simulink model "atrias_HW_boom_nmSt_kinSw_v2"  (R2015a)
settings: Solver=ode4  StartTime=0.0  StopTime=inf  FixedStep=sample_time  RelTol=1e-3
values from neighbouring files (symbols this model uses):
  control_start_time = 15    [setParams.m]
  flag_CtrlMode = 0    [setParams.m]
  kinSw_alpha_start = 130*pi/180    (= 2.26892802759)    [setParams.m]
  kinSw_alpha_tgt = 70*pi/180    (= 1.2217304764)    [setParams.m]
  kinSw_t_start = 0.5    [setParams.m]
  poser_LLegAlp = (initial_l_leg_angle -pi/2)*180/pi    (= 105)    [setParams.m]
  poser_LLegLen = initial_l_leg_length    (= 0.8)    [setParams.m]
  poser_RLegAlp = (initial_r_leg_angle -pi/2)*180/pi    (= 75)    [setParams.m]
  poser_RLegLen = initial_r_leg_length    (= 0.8)    [setParams.m]
  tune_kinSw_alpha_start = kinSw_alpha_start*180/pi    (= 130)    [setParams.m]
  tune_kinSw_alpha_tgt = kinSw_alpha_tgt*180/pi    (= 70)    [setParams.m]
  tune_kinSw_len_min = kinSw_len_min    (= 0.6)    [setParams.m]
  tune_kinSw_len_tgt = kinSw_len_tgt    (= 0.9)    [setParams.m]
  tune_M1_G = 9.5    [setParams.m]
  tune_M3_0 = CtrlPar_theta0*180/pi    [setParams.m]
  tune_M3_D = St_GainDTh_HFL*5    [setParams.m]
  tune_M3_P = St_GainTh_HFL*5    [setParams.m]
undefined symbols (not defined in the file or in its folder): A1_notch_f1, A2_notch_f1, A_kalman_fourbar_gear, A_lpf_dtau, B1_lpf_dtau, B1_notch_f1, B2_lpf_dtau, B2_notch_f1, B_kalman_fourbar_gear, boom_mount_angle, boom_mount_to_center_diagonal, c_jointstop, C_kalman_fourbar_gear, contactThr, d_vertical_com, delta_phi_max, delta_phi_max_buffer, delta_phi_max_dropoff, delta_phi_min, Discrete, FmaxBFSH, FmaxGLU, FmaxHAM, FmaxHFL, FmaxRF, FmaxVAS, FPCtrlPar, g, gain_nodes_sea_torque, HIP_MTR_MAX_CONT_TORQUE, initial_dx_estimate, j_motor, k_leg_spring, K_notch_f1, k_sea, kalman_load_to_deflect_transmission, kd_lateral, kd_motor, kd_shin_max, kd_shin_min, kd_splay_max, kd_splay_min, kd_thigh_max, kd_thigh_min, kp_lateral, kp_motor, kp_sea_torque, kp_shin_max, kp_shin_min, kp_splay_max, kp_splay_min, kp_thigh_max, kp_thigh_min, l_boom, l_seg, l_v, lateral_motor_efficiency, lateral_offset, lateral_target_angle_right, lateral_transition_force ... (+124)
libraries: simulink_extras x27, simulink x11, ctrlSharedLib x4
(part 4 of 8)

== system atrias_HW_boom_nmSt_kinSw_v2/Control/Behavior Control/Virtual Neuromuscular Control/Muscle Layer/GLU1 ==
  note: SOLEUS Muscle-Tendon Dynamics
  note: Excitation Contraction Coupling
  STIM : Inport
  lmtc [m] : Inport  Port=2
  1 : Product  Inputs=**  SaturateOnIntegerOverflow=on  InputSameDT=on  OutDataTypeStr=Inherit: Same as first input
  1/lslack : Gain  Gain=1/lslackGLU  SaturateOnIntegerOverflow=on  OutDataTypeStr=Inherit: Same as input  ParamDataTypeStr=Inherit: Same as input
  BE force-length relation : Subsystem
  CE force-length relation : Subsystem
  CE inverse force-velocity relation : Subsystem
  Constant : Constant  Value=lslackGLU
  ECC TransferFcn : simulink_extras/Additional Linear/Transfer Fcn (with initial outputs)  N=[1]  D="[mtu_tau  1]"  Y0=mtu_preA  U0=0
      settings: AttributesFormatString=pre-activation: %<Y0>
  Fmax : Gain  Gain=FmaxGLU  SaturateOnIntegerOverflow=on  OutDataTypeStr=Inherit: Same as input  ParamDataTypeStr=Inherit: Same as input
  Fv = Fse / (A*Fce) : Product  Inputs=*/  SaturateOnIntegerOverflow=on  InputSameDT=on  OutDataTypeStr=Inherit: Same as first input
  Integrator : Integrator  InitialConditionSource=external  LowerSaturationLimit=0.05
  PE force-length relation : Subsystem
  SE force-length relation : Subsystem
  Saturation : Saturate  UpperLimit=1  LowerLimit=0.01
  Sum : Sum  Inputs=|+-  SaturateOnIntegerOverflow=on  InputSameDT=on  OutDataTypeStr=Inherit: Same as first input
  Sum2 : Sum  Inputs=|-+  SaturateOnIntegerOverflow=on  InputSameDT=on  OutDataTypeStr=Inherit: Same as first input
  Sum3 : Sum  SaturateOnIntegerOverflow=on  InputSameDT=on  OutDataTypeStr=Inherit: Same as first input
  Sum4 : Sum  SaturateOnIntegerOverflow=on  InputSameDT=on  OutDataTypeStr=Inherit: Same as first input
  lce/lopt : Gain  Gain=1/loptGLU  SaturateOnIntegerOverflow=on  OutDataTypeStr=Inherit: Same as input  ParamDataTypeStr=Inherit: Same as input
  vmax*lopt : Gain  Gain=vmaxGLU*loptGLU  SaturateOnIntegerOverflow=on  OutDataTypeStr=Inherit: Same as input  ParamDataTypeStr=Inherit: Same as input
  Fmtc : Outport  InitialOutput=0
  Lce : Outport  Port=2  InitialOutput=0
  Vce : Outport  Port=3  InitialOutput=0
  A : Outport  Port=4  InitialOutput=0
  wires:
  Integrator/1 -> Sum/2, lce/lopt/1, Lce/1  "lce"
  Sum/1 -> 1/lslack/1  "lse"
  lce/lopt/1 -> CE force-length relation/1(lce [lopt]), BE force-length relation/1(lce [lopt]), PE force-length relation/1(lce [lopt])
  Fv = Fse / (A*Fce)/1 -> CE inverse force-velocity relation/1(Fv[Fmax])  "fv"
  vmax*lopt/1 -> Integrator/1, Vce/1  "vce"
  lmtc [m]/1 -> Sum2/2, Sum/1  "lmtc"
  Fmax/1 -> Fmtc/1  "Fmtc"
  1/lslack/1 -> SE force-length relation/1(lse [lslack])
  SE force-length relation/1(fse [Fmax]) -> Fmax/1, Sum4/1
  Sum2/1 -> Integrator/2
  Constant/1 -> Sum2/1
  CE force-length relation/1(fce [Fmax]) -> 1/1
  Sum4/1 -> Fv = Fse / (A*Fce)/1
  PE force-length relation/1(fpe [Fmax]) -> Sum3/1
  1/1 -> Sum3/2
  BE force-length relation/1(fbe [Fmax]) -> Sum4/2
  Sum3/1 -> Fv = Fse / (A*Fce)/2
  CE inverse force-velocity relation/1(v[vmax]) -> vmax*lopt/1
  STIM/1 -> ECC TransferFcn/1
  ECC TransferFcn/1 -> Saturation/1
  Saturation/1 -> A/1, 1/2

== system atrias_HW_boom_nmSt_kinSw_v2/Control/Behavior Control/Virtual Neuromuscular Control/Muscle Layer/HAM ==
  note: SOLEUS Muscle-Tendon Dynamics
  note: Excitation Contraction Coupling
  STIM : Inport
  lmtc [m] : Inport  Port=2
  1 : Product  Inputs=**  SaturateOnIntegerOverflow=on  InputSameDT=on  OutDataTypeStr=Inherit: Same as first input
  1/lslack : Gain  Gain=1/lslackHAM  SaturateOnIntegerOverflow=on  OutDataTypeStr=Inherit: Same as input  ParamDataTypeStr=Inherit: Same as input
  BE force-length relation : Subsystem
  CE force-length relation : Subsystem
  CE inverse force-velocity relation : Subsystem
  Constant : Constant  Value=lslackHAM
  ECC TransferFcn : simulink_extras/Additional Linear/Transfer Fcn (with initial outputs)  N=[1]  D="[mtu_tau  1]"  Y0=mtu_preA  U0=0
      settings: AttributesFormatString=pre-activation: %<Y0>
  Fmax : Gain  Gain=FmaxHAM  SaturateOnIntegerOverflow=on  OutDataTypeStr=Inherit: Same as input  ParamDataTypeStr=Inherit: Same as input
  Fv = Fse / (A*Fce) : Product  Inputs=*/  SaturateOnIntegerOverflow=on  InputSameDT=on  OutDataTypeStr=Inherit: Same as first input
  Integrator : Integrator  InitialConditionSource=external  LowerSaturationLimit=0.05
  PE force-length relation : Subsystem
  SE force-length relation : Subsystem
  Saturation : Saturate  UpperLimit=1  LowerLimit=0.01
  Sum : Sum  Inputs=|+-  SaturateOnIntegerOverflow=on  InputSameDT=on  OutDataTypeStr=Inherit: Same as first input
  Sum2 : Sum  Inputs=|-+  SaturateOnIntegerOverflow=on  InputSameDT=on  OutDataTypeStr=Inherit: Same as first input
  Sum3 : Sum  SaturateOnIntegerOverflow=on  InputSameDT=on  OutDataTypeStr=Inherit: Same as first input
  Sum4 : Sum  SaturateOnIntegerOverflow=on  InputSameDT=on  OutDataTypeStr=Inherit: Same as first input
  lce/lopt : Gain  Gain=1/loptHAM  SaturateOnIntegerOverflow=on  OutDataTypeStr=Inherit: Same as input  ParamDataTypeStr=Inherit: Same as input
  vmax*lopt : Gain  Gain=vmaxHAM*loptHAM  SaturateOnIntegerOverflow=on  OutDataTypeStr=Inherit: Same as input  ParamDataTypeStr=Inherit: Same as input
  Fmtc : Outport  InitialOutput=0
  Lce : Outport  Port=2  InitialOutput=0
  Vce : Outport  Port=3  InitialOutput=0
  A : Outport  Port=4  InitialOutput=0
  wires:
  Integrator/1 -> Sum/2, lce/lopt/1, Lce/1  "lce"
  Sum/1 -> 1/lslack/1  "lse"
  lce/lopt/1 -> CE force-length relation/1(lce [lopt]), BE force-length relation/1(lce [lopt]), PE force-length relation/1(lce [lopt])
  Fv = Fse / (A*Fce)/1 -> CE inverse force-velocity relation/1(Fv[Fmax])  "fv"
  vmax*lopt/1 -> Integrator/1, Vce/1  "vce"
  lmtc [m]/1 -> Sum2/2, Sum/1  "lmtc"
  Fmax/1 -> Fmtc/1  "Fmtc"
  1/lslack/1 -> SE force-length relation/1(lse [lslack])
  SE force-length relation/1(fse [Fmax]) -> Fmax/1, Sum4/1
  Sum2/1 -> Integrator/2
  Constant/1 -> Sum2/1
  CE force-length relation/1(fce [Fmax]) -> 1/1
  Sum4/1 -> Fv = Fse / (A*Fce)/1
  PE force-length relation/1(fpe [Fmax]) -> Sum3/1
  1/1 -> Sum3/2
  BE force-length relation/1(fbe [Fmax]) -> Sum4/2
  Sum3/1 -> Fv = Fse / (A*Fce)/2
  CE inverse force-velocity relation/1(v[vmax]) -> vmax*lopt/1
  STIM/1 -> ECC TransferFcn/1
  ECC TransferFcn/1 -> Saturation/1
  Saturation/1 -> A/1, 1/2

== system atrias_HW_boom_nmSt_kinSw_v2/Control/Behavior Control/Virtual Neuromuscular Control/Muscle Layer/HAM Link ==
  note: HAM Attachment
  phi34 [rad] : Inport
  phi23 [rad] : Inport  Port=2
  Constant1 : Constant  Value=rHAMk
  Constant2 : Constant  Value=phirefHAMk
  Constant3 : Constant  Value=rHAMh
  Constant4 : Constant  Value=lslackHAM+loptHAM
  Constant5 : Constant  Value=phirefHAMh
  Gain2 : Gain  Gain=rhoHAMh
  Gain4 : Gain  Gain=rhoHAMk
  Product : Product  RndMeth=Zero
  Product1 : Product  RndMeth=Zero
  Sum1 : Sum  Inputs=|+-
  Sum4 : Sum  Inputs=|+-
  Sum5 : Sum  Inputs=-++
  lmtu [m] : Outport
  lever34 [m] : Outport  Port=2
  lever23 [m] : Outport  Port=3
  wires:
  Sum5/1 -> lmtu [m]/1
  Constant4/1 -> Sum5/2
  Gain4/1 -> Sum5/3
  Gain2/1 -> Sum5/1
  phi34 [rad]/1 -> Sum4/1
  Constant5/1 -> Sum4/2
  Sum4/1 -> Product/1
  Constant3/1 -> Product/2, lever34 [m]/1
  Product/1 -> Gain2/1
  phi23 [rad]/1 -> Sum1/1
  Constant2/1 -> Sum1/2
  Sum1/1 -> Product1/1
  Constant1/1 -> Product1/2, lever23 [m]/1
  Product1/1 -> Gain4/1

== system atrias_HW_boom_nmSt_kinSw_v2/Control/Behavior Control/Virtual Neuromuscular Control/Muscle Layer/HAM Link1 ==
  note: HAM Attachment
  phi34 [rad] : Inport
  phi23 [rad] : Inport  Port=2
  Constant1 : Constant  Value=rHAMk
  Constant2 : Constant  Value=phirefHAMk
  Constant3 : Constant  Value=rHAMh
  Constant4 : Constant  Value=lslackHAM+loptHAM
  Constant5 : Constant  Value=phirefHAMh
  Gain2 : Gain  Gain=rhoHAMh
  Gain4 : Gain  Gain=rhoHAMk
  Product : Product  RndMeth=Zero
  Product1 : Product  RndMeth=Zero
  Sum1 : Sum  Inputs=|+-
  Sum4 : Sum  Inputs=|+-
  Sum5 : Sum  Inputs=-++
  lmtu [m] : Outport
  lever34 [m] : Outport  Port=2
  lever23 [m] : Outport  Port=3
  wires:
  Sum5/1 -> lmtu [m]/1
  Constant4/1 -> Sum5/2
  Gain4/1 -> Sum5/3
  Gain2/1 -> Sum5/1
  phi34 [rad]/1 -> Sum4/1
  Constant5/1 -> Sum4/2
  Sum4/1 -> Product/1
  Constant3/1 -> Product/2, lever34 [m]/1
  Product/1 -> Gain2/1
  phi23 [rad]/1 -> Sum1/1
  Constant2/1 -> Sum1/2
  Sum1/1 -> Product1/1
  Constant1/1 -> Product1/2, lever23 [m]/1
  Product1/1 -> Gain4/1

== system atrias_HW_boom_nmSt_kinSw_v2/Control/Behavior Control/Virtual Neuromuscular Control/Muscle Layer/HAM1 ==
  note: SOLEUS Muscle-Tendon Dynamics
  note: Excitation Contraction Coupling
  STIM : Inport
  lmtc [m] : Inport  Port=2
  1 : Product  Inputs=**  SaturateOnIntegerOverflow=on  InputSameDT=on  OutDataTypeStr=Inherit: Same as first input
  1/lslack : Gain  Gain=1/lslackHAM  SaturateOnIntegerOverflow=on  OutDataTypeStr=Inherit: Same as input  ParamDataTypeStr=Inherit: Same as input
  BE force-length relation : Subsystem
  CE force-length relation : Subsystem
  CE inverse force-velocity relation : Subsystem
  Constant : Constant  Value=lslackHAM
  ECC TransferFcn : simulink_extras/Additional Linear/Transfer Fcn (with initial outputs)  N=[1]  D="[mtu_tau  1]"  Y0=mtu_preA  U0=0
      settings: AttributesFormatString=pre-activation: %<Y0>
  Fmax : Gain  Gain=FmaxHAM  SaturateOnIntegerOverflow=on  OutDataTypeStr=Inherit: Same as input  ParamDataTypeStr=Inherit: Same as input
  Fv = Fse / (A*Fce) : Product  Inputs=*/  SaturateOnIntegerOverflow=on  InputSameDT=on  OutDataTypeStr=Inherit: Same as first input
  Integrator : Integrator  InitialConditionSource=external  LowerSaturationLimit=0.05
  PE force-length relation : Subsystem
  SE force-length relation : Subsystem
  Saturation : Saturate  UpperLimit=1  LowerLimit=0.01
  Sum : Sum  Inputs=|+-  SaturateOnIntegerOverflow=on  InputSameDT=on  OutDataTypeStr=Inherit: Same as first input
  Sum2 : Sum  Inputs=|-+  SaturateOnIntegerOverflow=on  InputSameDT=on  OutDataTypeStr=Inherit: Same as first input
  Sum3 : Sum  SaturateOnIntegerOverflow=on  InputSameDT=on  OutDataTypeStr=Inherit: Same as first input
  Sum4 : Sum  SaturateOnIntegerOverflow=on  InputSameDT=on  OutDataTypeStr=Inherit: Same as first input
  lce/lopt : Gain  Gain=1/loptHAM  SaturateOnIntegerOverflow=on  OutDataTypeStr=Inherit: Same as input  ParamDataTypeStr=Inherit: Same as input
  vmax*lopt : Gain  Gain=vmaxHAM*loptHAM  SaturateOnIntegerOverflow=on  OutDataTypeStr=Inherit: Same as input  ParamDataTypeStr=Inherit: Same as input
  Fmtc : Outport  InitialOutput=0
  Lce : Outport  Port=2  InitialOutput=0
  Vce : Outport  Port=3  InitialOutput=0
  A : Outport  Port=4  InitialOutput=0
  wires:
  Integrator/1 -> Sum/2, lce/lopt/1, Lce/1  "lce"
  Sum/1 -> 1/lslack/1  "lse"
  lce/lopt/1 -> CE force-length relation/1(lce [lopt]), BE force-length relation/1(lce [lopt]), PE force-length relation/1(lce [lopt])
  Fv = Fse / (A*Fce)/1 -> CE inverse force-velocity relation/1(Fv[Fmax])  "fv"
  vmax*lopt/1 -> Integrator/1, Vce/1  "vce"
  lmtc [m]/1 -> Sum2/2, Sum/1  "lmtc"
  Fmax/1 -> Fmtc/1  "Fmtc"
  1/lslack/1 -> SE force-length relation/1(lse [lslack])
  SE force-length relation/1(fse [Fmax]) -> Fmax/1, Sum4/1
  Sum2/1 -> Integrator/2
  Constant/1 -> Sum2/1
  CE force-length relation/1(fce [Fmax]) -> 1/1
  Sum4/1 -> Fv = Fse / (A*Fce)/1
  PE force-length relation/1(fpe [Fmax]) -> Sum3/1
  1/1 -> Sum3/2
  BE force-length relation/1(fbe [Fmax]) -> Sum4/2
  Sum3/1 -> Fv = Fse / (A*Fce)/2
  CE inverse force-velocity relation/1(v[vmax]) -> vmax*lopt/1
  STIM/1 -> ECC TransferFcn/1
  ECC TransferFcn/1 -> Saturation/1
  Saturation/1 -> A/1, 1/2

== system atrias_HW_boom_nmSt_kinSw_v2/Control/Behavior Control/Virtual Neuromuscular Control/Muscle Layer/HFL ==
  note: SOLEUS Muscle-Tendon Dynamics
  note: Excitation Contraction Coupling
  STIM : Inport
  lmtc [m] : Inport  Port=2
  1 : Product  Inputs=**  SaturateOnIntegerOverflow=on  InputSameDT=on  OutDataTypeStr=Inherit: Same as first input
  1/lslack : Gain  Gain=1/lslackHFL  SaturateOnIntegerOverflow=on  OutDataTypeStr=Inherit: Same as input  ParamDataTypeStr=Inherit: Same as input
  BE force-length relation : Subsystem
  CE force-length relation : Subsystem
  CE inverse force-velocity relation : Subsystem
  Constant : Constant  Value=lslackHFL
  ECC TransferFcn : simulink_extras/Additional Linear/Transfer Fcn (with initial outputs)  N=[1]  D="[mtu_tau  1]"  Y0=mtu_preA  U0=0
      settings: AttributesFormatString=pre-activation: %<Y0>
  Fmax : Gain  Gain=FmaxHFL  SaturateOnIntegerOverflow=on  OutDataTypeStr=Inherit: Same as input  ParamDataTypeStr=Inherit: Same as input
  Fv = Fse / (A*Fce) : Product  Inputs=*/  SaturateOnIntegerOverflow=on  InputSameDT=on  OutDataTypeStr=Inherit: Same as first input
  Integrator : Integrator  InitialConditionSource=external  LowerSaturationLimit=0.05
  PE force-length relation : Subsystem
  SE force-length relation : Subsystem
  Saturation : Saturate  UpperLimit=1  LowerLimit=0.01
  Sum : Sum  Inputs=|+-  SaturateOnIntegerOverflow=on  InputSameDT=on  OutDataTypeStr=Inherit: Same as first input
  Sum2 : Sum  Inputs=|-+  SaturateOnIntegerOverflow=on  InputSameDT=on  OutDataTypeStr=Inherit: Same as first input
  Sum3 : Sum  SaturateOnIntegerOverflow=on  InputSameDT=on  OutDataTypeStr=Inherit: Same as first input
  Sum4 : Sum  SaturateOnIntegerOverflow=on  InputSameDT=on  OutDataTypeStr=Inherit: Same as first input
  lce/lopt : Gain  Gain=1/loptHFL  SaturateOnIntegerOverflow=on  OutDataTypeStr=Inherit: Same as input  ParamDataTypeStr=Inherit: Same as input
  vmax*lopt : Gain  Gain=vmaxHFL*loptHFL  SaturateOnIntegerOverflow=on  OutDataTypeStr=Inherit: Same as input  ParamDataTypeStr=Inherit: Same as input
  Fmtc : Outport  InitialOutput=0
  Lce : Outport  Port=2  InitialOutput=0
  Vce : Outport  Port=3  InitialOutput=0
  A : Outport  Port=4  InitialOutput=0
  wires:
  Integrator/1 -> Sum/2, lce/lopt/1, Lce/1  "lce"
  Sum/1 -> 1/lslack/1  "lse"
  lce/lopt/1 -> CE force-length relation/1(lce [lopt]), BE force-length relation/1(lce [lopt]), PE force-length relation/1(lce [lopt])
  Fv = Fse / (A*Fce)/1 -> CE inverse force-velocity relation/1(Fv[Fmax])  "fv"
  vmax*lopt/1 -> Integrator/1, Vce/1  "vce"
  lmtc [m]/1 -> Sum2/2, Sum/1  "lmtc"
  Fmax/1 -> Fmtc/1  "Fmtc"
  1/lslack/1 -> SE force-length relation/1(lse [lslack])
  SE force-length relation/1(fse [Fmax]) -> Fmax/1, Sum4/1
  Sum2/1 -> Integrator/2
  Constant/1 -> Sum2/1
  CE force-length relation/1(fce [Fmax]) -> 1/1
  Sum4/1 -> Fv = Fse / (A*Fce)/1
  PE force-length relation/1(fpe [Fmax]) -> Sum3/1
  1/1 -> Sum3/2
  BE force-length relation/1(fbe [Fmax]) -> Sum4/2
  Sum3/1 -> Fv = Fse / (A*Fce)/2
  CE inverse force-velocity relation/1(v[vmax]) -> vmax*lopt/1
  STIM/1 -> ECC TransferFcn/1
  ECC TransferFcn/1 -> Saturation/1
  Saturation/1 -> A/1, 1/2

== system atrias_HW_boom_nmSt_kinSw_v2/Control/Behavior Control/Virtual Neuromuscular Control/Muscle Layer/HFL Link ==
  note: HFL Attachment
  phi34 [rad] : Inport
  Constant : Constant  Value=lslackHFL+loptHFL
  Constant1 : Constant  Value=rHFL
  Constant2 : Constant  Value=phirefHFL
  Gain2 : Gain  Gain=rhoHFL
  Product : Product  RndMeth=Zero
  Sum2 : Sum  Inputs=|+-
  Sum5 : Sum  Inputs=|++
  lmtu [m] : Outport
  lever [m] : Outport  Port=2
  wires:
  Constant/1 -> Sum5/1
  Sum5/1 -> lmtu [m]/1
  Product/1 -> Gain2/1
  phi34 [rad]/1 -> Sum2/1
  Constant2/1 -> Sum2/2
  Sum2/1 -> Product/1
  Constant1/1 -> Product/2, lever [m]/1
  Gain2/1 -> Sum5/2

== system atrias_HW_boom_nmSt_kinSw_v2/Control/Behavior Control/Virtual Neuromuscular Control/Muscle Layer/HFL Link1 ==
  note: HFL Attachment
  phi34 [rad] : Inport
  Constant : Constant  Value=lslackHFL+loptHFL
  Constant1 : Constant  Value=rHFL
  Constant2 : Constant  Value=phirefHFL
  Gain2 : Gain  Gain=rhoHFL
  Product : Product  RndMeth=Zero
  Sum2 : Sum  Inputs=|+-
  Sum5 : Sum  Inputs=|++
  lmtu [m] : Outport
  lever [m] : Outport  Port=2
  wires:
  Constant/1 -> Sum5/1
  Sum5/1 -> lmtu [m]/1
  Product/1 -> Gain2/1
  phi34 [rad]/1 -> Sum2/1
  Constant2/1 -> Sum2/2
  Sum2/1 -> Product/1
  Constant1/1 -> Product/2, lever [m]/1
  Gain2/1 -> Sum5/2

== system atrias_HW_boom_nmSt_kinSw_v2/Control/Behavior Control/Virtual Neuromuscular Control/Muscle Layer/HFL1 ==
  note: SOLEUS Muscle-Tendon Dynamics
  note: Excitation Contraction Coupling
  STIM : Inport
  lmtc [m] : Inport  Port=2
  1 : Product  Inputs=**  SaturateOnIntegerOverflow=on  InputSameDT=on  OutDataTypeStr=Inherit: Same as first input
  1/lslack : Gain  Gain=1/lslackHFL  SaturateOnIntegerOverflow=on  OutDataTypeStr=Inherit: Same as input  ParamDataTypeStr=Inherit: Same as input
  BE force-length relation : Subsystem
  CE force-length relation : Subsystem
  CE inverse force-velocity relation : Subsystem
  Constant : Constant  Value=lslackHFL
  ECC TransferFcn : simulink_extras/Additional Linear/Transfer Fcn (with initial outputs)  N=[1]  D="[mtu_tau  1]"  Y0=mtu_preA  U0=0
      settings: AttributesFormatString=pre-activation: %<Y0>
  Fmax : Gain  Gain=FmaxHFL  SaturateOnIntegerOverflow=on  OutDataTypeStr=Inherit: Same as input  ParamDataTypeStr=Inherit: Same as input
  Fv = Fse / (A*Fce) : Product  Inputs=*/  SaturateOnIntegerOverflow=on  InputSameDT=on  OutDataTypeStr=Inherit: Same as first input
  Integrator : Integrator  InitialConditionSource=external  LowerSaturationLimit=0.05
  PE force-length relation : Subsystem
  SE force-length relation : Subsystem
  Saturation : Saturate  UpperLimit=1  LowerLimit=0.01
  Sum : Sum  Inputs=|+-  SaturateOnIntegerOverflow=on  InputSameDT=on  OutDataTypeStr=Inherit: Same as first input
  Sum2 : Sum  Inputs=|-+  SaturateOnIntegerOverflow=on  InputSameDT=on  OutDataTypeStr=Inherit: Same as first input
  Sum3 : Sum  SaturateOnIntegerOverflow=on  InputSameDT=on  OutDataTypeStr=Inherit: Same as first input
  Sum4 : Sum  SaturateOnIntegerOverflow=on  InputSameDT=on  OutDataTypeStr=Inherit: Same as first input
  lce/lopt : Gain  Gain=1/loptHFL  SaturateOnIntegerOverflow=on  OutDataTypeStr=Inherit: Same as input  ParamDataTypeStr=Inherit: Same as input
  vmax*lopt : Gain  Gain=vmaxHFL*loptHFL  SaturateOnIntegerOverflow=on  OutDataTypeStr=Inherit: Same as input  ParamDataTypeStr=Inherit: Same as input
  Fmtc : Outport  InitialOutput=0
  Lce : Outport  Port=2  InitialOutput=0
  Vce : Outport  Port=3  InitialOutput=0
  A : Outport  Port=4  InitialOutput=0
  wires:
  Integrator/1 -> Sum/2, lce/lopt/1, Lce/1  "lce"
  Sum/1 -> 1/lslack/1  "lse"
  lce/lopt/1 -> CE force-length relation/1(lce [lopt]), BE force-length relation/1(lce [lopt]), PE force-length relation/1(lce [lopt])
  Fv = Fse / (A*Fce)/1 -> CE inverse force-velocity relation/1(Fv[Fmax])  "fv"
  vmax*lopt/1 -> Integrator/1, Vce/1  "vce"
  lmtc [m]/1 -> Sum2/2, Sum/1  "lmtc"
  Fmax/1 -> Fmtc/1  "Fmtc"
  1/lslack/1 -> SE force-length relation/1(lse [lslack])
  SE force-length relation/1(fse [Fmax]) -> Fmax/1, Sum4/1
  Sum2/1 -> Integrator/2
  Constant/1 -> Sum2/1
  CE force-length relation/1(fce [Fmax]) -> 1/1
  Sum4/1 -> Fv = Fse / (A*Fce)/1
  PE force-length relation/1(fpe [Fmax]) -> Sum3/1
  1/1 -> Sum3/2
  BE force-length relation/1(fbe [Fmax]) -> Sum4/2
  Sum3/1 -> Fv = Fse / (A*Fce)/2
  CE inverse force-velocity relation/1(v[vmax]) -> vmax*lopt/1
  STIM/1 -> ECC TransferFcn/1
  ECC TransferFcn/1 -> Saturation/1
  Saturation/1 -> A/1, 1/2

== system atrias_HW_boom_nmSt_kinSw_v2/Control/Behavior Control/Virtual Neuromuscular Control/Muscle Layer/L BFSH Link ==
  note: BFSH Attachment
  phi23 [rad] : Inport
  Constant : Constant  Value=lslackBFSH+loptBFSH
  Constant1 : Constant  Value=rBFSH
  Constant2 : Constant  Value=phirefBFSH
  Gain4 : Gain  Gain=rhoBFSH
  Product : Product  RndMeth=Zero
  Sum2 : Sum  Inputs=|+-
  Sum5 : Sum  Inputs=|++
  lmtu [m] : Outport
  lever [m] : Outport  Port=2
  wires:
  Constant/1 -> Sum5/1
  Sum5/1 -> lmtu [m]/1
  Gain4/1 -> Sum5/2
  Product/1 -> Gain4/1
  phi23 [rad]/1 -> Sum2/1
  Constant2/1 -> Sum2/2
  Sum2/1 -> Product/1
  Constant1/1 -> Product/2, lever [m]/1

== system atrias_HW_boom_nmSt_kinSw_v2/Control/Behavior Control/Virtual Neuromuscular Control/Muscle Layer/L BFSH Link1 ==
  note: BFSH Attachment
  phi23 [rad] : Inport
  Constant : Constant  Value=lslackBFSH+loptBFSH
  Constant1 : Constant  Value=rBFSH
  Constant2 : Constant  Value=phirefBFSH
  Gain4 : Gain  Gain=rhoBFSH
  Product : Product  RndMeth=Zero
  Sum2 : Sum  Inputs=|+-
  Sum5 : Sum  Inputs=|++
  lmtu [m] : Outport
  lever [m] : Outport  Port=2
  wires:
  Constant/1 -> Sum5/1
  Sum5/1 -> lmtu [m]/1
  Gain4/1 -> Sum5/2
  Product/1 -> Gain4/1
  phi23 [rad]/1 -> Sum2/1
  Constant2/1 -> Sum2/2
  Sum2/1 -> Product/1
  Constant1/1 -> Product/2, lever [m]/1

== system atrias_HW_boom_nmSt_kinSw_v2/Control/Behavior Control/Virtual Neuromuscular Control/Muscle Layer/L Hip Joint Limits ==
  note: Hip Joint Limits
  phi [rad]1 : Inport
  dphi [rad/s]1 : Inport  Port=2
  Constant : Constant  Value=0
  Gain1 : Gain  Gain=c_jointstop
  Gain5 : Gain  Gain=-1
  Gain6 : Gain  Gain=c_jointstop
  Gain7 : Gain  Gain=1/w_max_jointstop
  Manual Switch : ManualSwitch
  Mux1 : Mux  Inputs=2
  Mux2 : Mux  Inputs=2
  Overextension Torque1 : Fcn  Expr="- u(1)  *  (1-u(2)) * (u(2)<1) * (u(1)>0)"
  Overflexion Torque : Fcn  Expr="- u(1)  *  (1-u(2)) * (u(2)<1) * (u(1)<0)"
  Sum1 : Sum  Inputs=|+-
  Sum2 : Sum  Inputs=|+-
  Sum3 : Sum
  overextension angle1 : Constant  Value=phi23_max
  overflexion angle : Constant  Value=phi23_min
  M_stop [Nm]1 : Outport
  wires:
  Mux2/1 -> Overextension Torque1/1
  Gain6/1 -> Mux2/1
  dphi [rad/s]1/1 -> Gain7/1
  overextension angle1/1 -> Sum1/2
  phi [rad]1/1 -> Sum1/1, Sum2/1
  Sum1/1 -> Gain6/1
  Gain7/1 -> Gain5/1, Mux1/2
  Gain1/1 -> Mux1/1
  Sum2/1 -> Gain1/1
  overflexion angle/1 -> Sum2/2
  Mux1/1 -> Overflexion Torque/1
  Gain5/1 -> Mux2/2
  Overflexion Torque/1 -> Sum3/2
  Overextension Torque1/1 -> Sum3/1
  Sum3/1 -> Manual Switch/1
  Constant/1 -> Manual Switch/2
  Manual Switch/1 -> M_stop [Nm]1/1

== system atrias_HW_boom_nmSt_kinSw_v2/Control/Behavior Control/Virtual Neuromuscular Control/Muscle Layer/L Hip Joint Limits1 ==
  note: Hip Joint Limits
  phi [rad]1 : Inport
  dphi [rad/s]1 : Inport  Port=2
  Constant : Constant  Value=0
  Gain1 : Gain  Gain=c_jointstop
  Gain5 : Gain  Gain=-1
  Gain6 : Gain  Gain=c_jointstop
  Gain7 : Gain  Gain=1/w_max_jointstop
  Manual Switch : ManualSwitch
  Mux1 : Mux  Inputs=2
  Mux2 : Mux  Inputs=2
  Overextension Torque1 : Fcn  Expr="- u(1)  *  (1-u(2)) * (u(2)<1) * (u(1)>0)"
  Overflexion Torque : Fcn  Expr="- u(1)  *  (1-u(2)) * (u(2)<1) * (u(1)<0)"
  Sum1 : Sum  Inputs=|+-
  Sum2 : Sum  Inputs=|+-
  Sum3 : Sum
  overextension angle1 : Constant  Value=phi23_max
  overflexion angle : Constant  Value=phi23_min
  M_stop [Nm]1 : Outport
  wires:
  Mux2/1 -> Overextension Torque1/1
  Gain6/1 -> Mux2/1
  dphi [rad/s]1/1 -> Gain7/1
  overextension angle1/1 -> Sum1/2
  phi [rad]1/1 -> Sum1/1, Sum2/1
  Sum1/1 -> Gain6/1
  Gain7/1 -> Gain5/1, Mux1/2
  Gain1/1 -> Mux1/1
  Sum2/1 -> Gain1/1
  overflexion angle/1 -> Sum2/2
  Mux1/1 -> Overflexion Torque/1
  Gain5/1 -> Mux2/2
  Overflexion Torque/1 -> Sum3/2
  Overextension Torque1/1 -> Sum3/1
  Sum3/1 -> Manual Switch/1
  Constant/1 -> Manual Switch/2
  Manual Switch/1 -> M_stop [Nm]1/1

== system atrias_HW_boom_nmSt_kinSw_v2/Control/Behavior Control/Virtual Neuromuscular Control/Muscle Layer/L Knee Joint Limits ==
  note: Knee Joint Limits
  phi [rad]1 : Inport
  dphi [rad/s]1 : Inport  Port=2
  Constant : Constant  Value=0
  Gain1 : Gain  Gain=c_jointstop
  Gain5 : Gain  Gain=-1
  Gain6 : Gain  Gain=c_jointstop
  Gain7 : Gain  Gain=1/w_max_jointstop
  Manual Switch : ManualSwitch
  Mux1 : Mux  Inputs=2
  Mux2 : Mux  Inputs=2
  Overextension Torque1 : Fcn  Expr="- u(1)  *  (1-u(2)) * (u(2)<1) * (u(1)>0)"
  Overflexion Torque : Fcn  Expr="- u(1)  *  (1-u(2)) * (u(2)<1) * (u(1)<0)"
  Sum1 : Sum  Inputs=|+-
  Sum2 : Sum  Inputs=|+-
  Sum3 : Sum
  overextension angle1 : Constant  Value=phi12_max
  overflexion angle : Constant  Value=phi12_min
  M_stop [Nm]1 : Outport
  wires:
  Mux2/1 -> Overextension Torque1/1
  Gain6/1 -> Mux2/1
  dphi [rad/s]1/1 -> Gain7/1
  overextension angle1/1 -> Sum1/2
  phi [rad]1/1 -> Sum1/1, Sum2/1
  Sum1/1 -> Gain6/1
  Gain7/1 -> Gain5/1, Mux1/2
  Gain1/1 -> Mux1/1
  Sum2/1 -> Gain1/1
  overflexion angle/1 -> Sum2/2
  Mux1/1 -> Overflexion Torque/1
  Gain5/1 -> Mux2/2
  Overflexion Torque/1 -> Sum3/2
  Overextension Torque1/1 -> Sum3/1
  Sum3/1 -> Manual Switch/1
  Constant/1 -> Manual Switch/2
  Manual Switch/1 -> M_stop [Nm]1/1

== system atrias_HW_boom_nmSt_kinSw_v2/Control/Behavior Control/Virtual Neuromuscular Control/Muscle Layer/L Knee Joint Limits1 ==
  note: Knee Joint Limits
  phi [rad]1 : Inport
  dphi [rad/s]1 : Inport  Port=2
  Constant : Constant  Value=0
  Gain1 : Gain  Gain=c_jointstop
  Gain5 : Gain  Gain=-1
  Gain6 : Gain  Gain=c_jointstop
  Gain7 : Gain  Gain=1/w_max_jointstop
  Manual Switch : ManualSwitch
  Mux1 : Mux  Inputs=2
  Mux2 : Mux  Inputs=2
  Overextension Torque1 : Fcn  Expr="- u(1)  *  (1-u(2)) * (u(2)<1) * (u(1)>0)"
  Overflexion Torque : Fcn  Expr="- u(1)  *  (1-u(2)) * (u(2)<1) * (u(1)<0)"
  Sum1 : Sum  Inputs=|+-
  Sum2 : Sum  Inputs=|+-
  Sum3 : Sum
  overextension angle1 : Constant  Value=phi12_max
  overflexion angle : Constant  Value=phi12_min
  M_stop [Nm]1 : Outport
  wires:
  Mux2/1 -> Overextension Torque1/1
  Gain6/1 -> Mux2/1
  dphi [rad/s]1/1 -> Gain7/1
  overextension angle1/1 -> Sum1/2
  phi [rad]1/1 -> Sum1/1, Sum2/1
  Sum1/1 -> Gain6/1
  Gain7/1 -> Gain5/1, Mux1/2
  Gain1/1 -> Mux1/1
  Sum2/1 -> Gain1/1
  overflexion angle/1 -> Sum2/2
  Mux1/1 -> Overflexion Torque/1
  Gain5/1 -> Mux2/2
  Overflexion Torque/1 -> Sum3/2
  Overextension Torque1/1 -> Sum3/1
  Sum3/1 -> Manual Switch/1
  Constant/1 -> Manual Switch/2
  Manual Switch/1 -> M_stop [Nm]1/1

== system atrias_HW_boom_nmSt_kinSw_v2/Control/Behavior Control/Virtual Neuromuscular Control/Muscle Layer/RF ==
  note: SOLEUS Muscle-Tendon Dynamics
  note: Excitation Contraction Coupling
  STIM : Inport
  lmtc [m] : Inport  Port=2
  1 : Product  Inputs=**  SaturateOnIntegerOverflow=on  InputSameDT=on  OutDataTypeStr=Inherit: Same as first input
  1/lslack : Gain  Gain=1/lslackRF  SaturateOnIntegerOverflow=on  OutDataTypeStr=Inherit: Same as input  ParamDataTypeStr=Inherit: Same as input
  BE force-length relation : Subsystem
  CE force-length relation : Subsystem
  CE inverse force-velocity relation : Subsystem
  Constant : Constant  Value=lslackRF
  ECC TransferFcn : simulink_extras/Additional Linear/Transfer Fcn (with initial outputs)  N=[1]  D="[mtu_tau  1]"  Y0=mtu_preA  U0=0
      settings: AttributesFormatString=pre-activation: %<Y0>
  Fmax : Gain  Gain=FmaxRF  SaturateOnIntegerOverflow=on  OutDataTypeStr=Inherit: Same as input  ParamDataTypeStr=Inherit: Same as input
  Fv = Fse / (A*Fce) : Product  Inputs=*/  SaturateOnIntegerOverflow=on  InputSameDT=on  OutDataTypeStr=Inherit: Same as first input
  Integrator : Integrator  InitialConditionSource=external  LowerSaturationLimit=0.05
  PE force-length relation : Subsystem
  SE force-length relation : Subsystem
  Saturation : Saturate  UpperLimit=1  LowerLimit=0.01
  Sum : Sum  Inputs=|+-  SaturateOnIntegerOverflow=on  InputSameDT=on  OutDataTypeStr=Inherit: Same as first input
  Sum2 : Sum  Inputs=|-+  SaturateOnIntegerOverflow=on  InputSameDT=on  OutDataTypeStr=Inherit: Same as first input
  Sum3 : Sum  SaturateOnIntegerOverflow=on  InputSameDT=on  OutDataTypeStr=Inherit: Same as first input
  Sum4 : Sum  SaturateOnIntegerOverflow=on  InputSameDT=on  OutDataTypeStr=Inherit: Same as first input
  lce/lopt : Gain  Gain=1/loptRF  SaturateOnIntegerOverflow=on  OutDataTypeStr=Inherit: Same as input  ParamDataTypeStr=Inherit: Same as input
  vmax*lopt : Gain  Gain=vmaxRF*loptRF  SaturateOnIntegerOverflow=on  OutDataTypeStr=Inherit: Same as input  ParamDataTypeStr=Inherit: Same as input
  Fmtc : Outport  InitialOutput=0
  Lce : Outport  Port=2  InitialOutput=0
  Vce : Outport  Port=3  InitialOutput=0
  A : Outport  Port=4  InitialOutput=0
  wires:
  Integrator/1 -> Sum/2, lce/lopt/1, Lce/1  "lce"
  Sum/1 -> 1/lslack/1  "lse"
  lce/lopt/1 -> CE force-length relation/1(lce [lopt]), BE force-length relation/1(lce [lopt]), PE force-length relation/1(lce [lopt])
  Fv = Fse / (A*Fce)/1 -> CE inverse force-velocity relation/1(Fv[Fmax])  "fv"
  vmax*lopt/1 -> Integrator/1, Vce/1  "vce"
  lmtc [m]/1 -> Sum2/2, Sum/1  "lmtc"
  Fmax/1 -> Fmtc/1  "Fmtc"
  1/lslack/1 -> SE force-length relation/1(lse [lslack])
  SE force-length relation/1(fse [Fmax]) -> Fmax/1, Sum4/1
  Sum2/1 -> Integrator/2
  Constant/1 -> Sum2/1
  CE force-length relation/1(fce [Fmax]) -> 1/1
  Sum4/1 -> Fv = Fse / (A*Fce)/1
  PE force-length relation/1(fpe [Fmax]) -> Sum3/1
  1/1 -> Sum3/2
  BE force-length relation/1(fbe [Fmax]) -> Sum4/2
  Sum3/1 -> Fv = Fse / (A*Fce)/2
  CE inverse force-velocity relation/1(v[vmax]) -> vmax*lopt/1
  STIM/1 -> ECC TransferFcn/1
  ECC TransferFcn/1 -> Saturation/1
  Saturation/1 -> A/1, 1/2

== system atrias_HW_boom_nmSt_kinSw_v2/Control/Behavior Control/Virtual Neuromuscular Control/Muscle Layer/RF Link ==
  note: RF Attachment
  phi34 [rad] : Inport
  phi23 [rad] : Inport  Port=2
  Constant1 : Constant  Value=phimaxRFk
  Constant2 : Constant  Value=phirefRFk
  Constant3 : Constant  Value=rRFh
  Constant4 : Constant  Value=lslackRF+loptRF
  Constant5 : Constant  Value=phirefRFh
  Demux : Demux  Outputs=2
  Display : Display
  Gain1 : Gain  Gain=rRFkmax
  Gain2 : Gain  Gain=rhoRFh
  Gain3 : Gain  Gain=phiScaleRFk
  Gain4 : Gain  Gain=rhoRFk/phiScaleRFk
  Gain5 : Gain  Gain=phiScaleRFk
  Mux : Mux  Inputs=2
  Product : Product  RndMeth=Zero
  Sum1 : Sum  Inputs=-+
  Sum2 : Sum  Inputs=|+-
  Sum3 : Sum  Inputs=-+|
  Sum4 : Sum  Inputs=|+-
  Sum5 : Sum  Inputs=++-
  length change term : Trigonometry
  offset correction term : Trigonometry
  variable lever term : Trigonometry  Operator=cos
  lmtu [m] : Outport
  lever34 [m] : Outport  Port=2
  lever23 [m] : Outport  Port=3
  wires:
  Sum5/1 -> Display/1, lmtu [m]/1
  Constant4/1 -> Sum5/2
  Gain4/1 -> Sum5/3
  Gain2/1 -> Sum5/1
  phi34 [rad]/1 -> Sum4/1
  Constant5/1 -> Sum4/2
  Sum4/1 -> Product/1
  Constant3/1 -> Product/2, lever34 [m]/1
  Product/1 -> Gain2/1
  phi23 [rad]/1 -> Sum3/2
  Sum3/1 -> Gain3/1
  Constant1/1 -> Sum3/1, Sum2/2
  Sum2/1 -> Gain5/1
  Constant2/1 -> Sum2/1
  length change term/1 -> Sum1/2
  offset correction term/1 -> Sum1/1
  Sum1/1 -> Mux/1
  variable lever term/1 -> Mux/2
  Mux/1 -> Gain1/1
  Gain1/1 -> Demux/1
  Demux/2 -> lever23 [m]/1
  Demux/1 -> Gain4/1
  Gain3/1 -> variable lever term/1, length change term/1
  Gain5/1 -> offset correction term/1

== system atrias_HW_boom_nmSt_kinSw_v2/Control/Behavior Control/Virtual Neuromuscular Control/Muscle Layer/RF Link1 ==
  note: RF Attachment
  phi34 [rad] : Inport
  phi23 [rad] : Inport  Port=2
  Constant1 : Constant  Value=phimaxRFk
  Constant2 : Constant  Value=phirefRFk
  Constant3 : Constant  Value=rRFh
  Constant4 : Constant  Value=lslackRF+loptRF
  Constant5 : Constant  Value=phirefRFh
  Demux : Demux  Outputs=2
  Gain1 : Gain  Gain=rRFkmax
  Gain2 : Gain  Gain=rhoRFh
  Gain3 : Gain  Gain=phiScaleRFk
  Gain4 : Gain  Gain=rhoRFk/phiScaleRFk
  Gain5 : Gain  Gain=phiScaleRFk
  Mux : Mux  Inputs=2
  Product : Product  RndMeth=Zero
  Sum1 : Sum  Inputs=-+
  Sum2 : Sum  Inputs=|+-
  Sum3 : Sum  Inputs=-+|
  Sum4 : Sum  Inputs=|+-
  Sum5 : Sum  Inputs=++-
  length change term : Trigonometry
  offset correction term : Trigonometry
  variable lever term : Trigonometry  Operator=cos
  lmtu [m] : Outport
  lever34 [m] : Outport  Port=2
  lever23 [m] : Outport  Port=3
  wires:
  Sum5/1 -> lmtu [m]/1
  Constant4/1 -> Sum5/2
  Gain4/1 -> Sum5/3
  Gain2/1 -> Sum5/1
  phi34 [rad]/1 -> Sum4/1
  Constant5/1 -> Sum4/2
  Sum4/1 -> Product/1
  Constant3/1 -> Product/2, lever34 [m]/1
  Product/1 -> Gain2/1
  phi23 [rad]/1 -> Sum3/2
  Sum3/1 -> Gain3/1
  Constant1/1 -> Sum3/1, Sum2/2
  Sum2/1 -> Gain5/1
  Constant2/1 -> Sum2/1
  length change term/1 -> Sum1/2
  offset correction term/1 -> Sum1/1
  Sum1/1 -> Mux/1
  variable lever term/1 -> Mux/2
  Mux/1 -> Gain1/1
  Gain1/1 -> Demux/1
  Demux/2 -> lever23 [m]/1
  Demux/1 -> Gain4/1
  Gain3/1 -> variable lever term/1, length change term/1
  Gain5/1 -> offset correction term/1

== system atrias_HW_boom_nmSt_kinSw_v2/Control/Behavior Control/Virtual Neuromuscular Control/Muscle Layer/RF1 ==
  note: SOLEUS Muscle-Tendon Dynamics
  note: Excitation Contraction Coupling
  STIM : Inport
  lmtc [m] : Inport  Port=2
  1 : Product  Inputs=**  SaturateOnIntegerOverflow=on  InputSameDT=on  OutDataTypeStr=Inherit: Same as first input
  1/lslack : Gain  Gain=1/lslackRF  SaturateOnIntegerOverflow=on  OutDataTypeStr=Inherit: Same as input  ParamDataTypeStr=Inherit: Same as input
  BE force-length relation : Subsystem
  CE force-length relation : Subsystem
  CE inverse force-velocity relation : Subsystem
  Constant : Constant  Value=lslackRF
  ECC TransferFcn : simulink_extras/Additional Linear/Transfer Fcn (with initial outputs)  N=[1]  D="[mtu_tau  1]"  Y0=mtu_preA  U0=0
      settings: AttributesFormatString=pre-activation: %<Y0>
  Fmax : Gain  Gain=FmaxRF  SaturateOnIntegerOverflow=on  OutDataTypeStr=Inherit: Same as input  ParamDataTypeStr=Inherit: Same as input
  Fv = Fse / (A*Fce) : Product  Inputs=*/  SaturateOnIntegerOverflow=on  InputSameDT=on  OutDataTypeStr=Inherit: Same as first input
  Integrator : Integrator  InitialConditionSource=external  LowerSaturationLimit=0.05
  PE force-length relation : Subsystem
  SE force-length relation : Subsystem
  Saturation : Saturate  UpperLimit=1  LowerLimit=0.01
  Sum : Sum  Inputs=|+-  SaturateOnIntegerOverflow=on  InputSameDT=on  OutDataTypeStr=Inherit: Same as first input
  Sum2 : Sum  Inputs=|-+  SaturateOnIntegerOverflow=on  InputSameDT=on  OutDataTypeStr=Inherit: Same as first input
  Sum3 : Sum  SaturateOnIntegerOverflow=on  InputSameDT=on  OutDataTypeStr=Inherit: Same as first input
  Sum4 : Sum  SaturateOnIntegerOverflow=on  InputSameDT=on  OutDataTypeStr=Inherit: Same as first input
  lce/lopt : Gain  Gain=1/loptRF  SaturateOnIntegerOverflow=on  OutDataTypeStr=Inherit: Same as input  ParamDataTypeStr=Inherit: Same as input
  vmax*lopt : Gain  Gain=vmaxRF*loptRF  SaturateOnIntegerOverflow=on  OutDataTypeStr=Inherit: Same as input  ParamDataTypeStr=Inherit: Same as input
  Fmtc : Outport  InitialOutput=0
  Lce : Outport  Port=2  InitialOutput=0
  Vce : Outport  Port=3  InitialOutput=0
  A : Outport  Port=4  InitialOutput=0
  wires:
  Integrator/1 -> Sum/2, lce/lopt/1, Lce/1  "lce"
  Sum/1 -> 1/lslack/1  "lse"
  lce/lopt/1 -> CE force-length relation/1(lce [lopt]), BE force-length relation/1(lce [lopt]), PE force-length relation/1(lce [lopt])
  Fv = Fse / (A*Fce)/1 -> CE inverse force-velocity relation/1(Fv[Fmax])  "fv"
  vmax*lopt/1 -> Integrator/1, Vce/1  "vce"
  lmtc [m]/1 -> Sum2/2, Sum/1  "lmtc"
  Fmax/1 -> Fmtc/1  "Fmtc"
  1/lslack/1 -> SE force-length relation/1(lse [lslack])
  SE force-length relation/1(fse [Fmax]) -> Fmax/1, Sum4/1
  Sum2/1 -> Integrator/2
  Constant/1 -> Sum2/1
  CE force-length relation/1(fce [Fmax]) -> 1/1
  Sum4/1 -> Fv = Fse / (A*Fce)/1
  PE force-length relation/1(fpe [Fmax]) -> Sum3/1
  1/1 -> Sum3/2
  BE force-length relation/1(fbe [Fmax]) -> Sum4/2
  Sum3/1 -> Fv = Fse / (A*Fce)/2
  CE inverse force-velocity relation/1(v[vmax]) -> vmax*lopt/1
  STIM/1 -> ECC TransferFcn/1
  ECC TransferFcn/1 -> Saturation/1
  Saturation/1 -> A/1, 1/2

== system atrias_HW_boom_nmSt_kinSw_v2/Control/Behavior Control/Virtual Neuromuscular Control/Muscle Layer/VAS ==
  note: SOLEUS Muscle-Tendon Dynamics
  note: Excitation Contraction Coupling
  STIM : Inport
  lmtc [m] : Inport  Port=2
  1 : Product  Inputs=**  SaturateOnIntegerOverflow=on  InputSameDT=on  OutDataTypeStr=Inherit: Same as first input
  1/lslack : Gain  Gain=1/lslackVAS  SaturateOnIntegerOverflow=on  OutDataTypeStr=Inherit: Same as input  ParamDataTypeStr=Inherit: Same as input
  BE force-length relation : Subsystem
  CE force-length relation : Subsystem
  CE inverse force-velocity relation : Subsystem
  Constant : Constant  Value=lslackVAS
  ECC TransferFcn : simulink_extras/Additional Linear/Transfer Fcn (with initial outputs)  N=[1]  D="[mtu_tau  1]"  Y0=mtu_preA  U0=0
      settings: AttributesFormatString=pre-activation: %<Y0>
  Fmax : Gain  Gain=FmaxVAS  SaturateOnIntegerOverflow=on  OutDataTypeStr=Inherit: Same as input  ParamDataTypeStr=Inherit: Same as input
  Fv = Fse / (A*Fce) : Product  Inputs=*/  SaturateOnIntegerOverflow=on  InputSameDT=on  OutDataTypeStr=Inherit: Same as first input
  Integrator : Integrator  InitialConditionSource=external  LowerSaturationLimit=0.05
  PE force-length relation : Subsystem
  SE force-length relation : Subsystem
  Saturation : Saturate  UpperLimit=1  LowerLimit=0.01
  Sum : Sum  Inputs=|+-  SaturateOnIntegerOverflow=on  InputSameDT=on  OutDataTypeStr=Inherit: Same as first input
  Sum2 : Sum  Inputs=|-+  SaturateOnIntegerOverflow=on  InputSameDT=on  OutDataTypeStr=Inherit: Same as first input
  Sum3 : Sum  SaturateOnIntegerOverflow=on  InputSameDT=on  OutDataTypeStr=Inherit: Same as first input
  Sum4 : Sum  SaturateOnIntegerOverflow=on  InputSameDT=on  OutDataTypeStr=Inherit: Same as first input
  lce/lopt : Gain  Gain=1/loptVAS  SaturateOnIntegerOverflow=on  OutDataTypeStr=Inherit: Same as input  ParamDataTypeStr=Inherit: Same as input
  vmax*lopt : Gain  Gain=vmaxVAS*loptVAS  SaturateOnIntegerOverflow=on  OutDataTypeStr=Inherit: Same as input  ParamDataTypeStr=Inherit: Same as input
  Fmtc : Outport  InitialOutput=0
  Lce : Outport  Port=2  InitialOutput=0
  Vce : Outport  Port=3  InitialOutput=0
  A : Outport  Port=4  InitialOutput=0
  wires:
  Integrator/1 -> Sum/2, lce/lopt/1, Lce/1  "lce"
  Sum/1 -> 1/lslack/1  "lse"
  lce/lopt/1 -> CE force-length relation/1(lce [lopt]), BE force-length relation/1(lce [lopt]), PE force-length relation/1(lce [lopt])
  Fv = Fse / (A*Fce)/1 -> CE inverse force-velocity relation/1(Fv[Fmax])  "fv"
  vmax*lopt/1 -> Integrator/1, Vce/1  "vce"
  lmtc [m]/1 -> Sum2/2, Sum/1  "lmtc"
  Fmax/1 -> Fmtc/1  "Fmtc"
  1/lslack/1 -> SE force-length relation/1(lse [lslack])
  SE force-length relation/1(fse [Fmax]) -> Fmax/1, Sum4/1
  Sum2/1 -> Integrator/2
  Constant/1 -> Sum2/1
  CE force-length relation/1(fce [Fmax]) -> 1/1
  Sum4/1 -> Fv = Fse / (A*Fce)/1
  PE force-length relation/1(fpe [Fmax]) -> Sum3/1
  1/1 -> Sum3/2
  BE force-length relation/1(fbe [Fmax]) -> Sum4/2
  Sum3/1 -> Fv = Fse / (A*Fce)/2
  CE inverse force-velocity relation/1(v[vmax]) -> vmax*lopt/1
  STIM/1 -> ECC TransferFcn/1
  ECC TransferFcn/1 -> Saturation/1
  Saturation/1 -> A/1, 1/2

== system atrias_HW_boom_nmSt_kinSw_v2/Control/Behavior Control/Virtual Neuromuscular Control/Muscle Layer/VAS Link ==
  note: Muscle Length and Moment Arm
  phi23 [rad] : Inport
  Constant : Constant  Value=lslackVAS+loptVAS
  Constant1 : Constant  Value=phimaxVAS
  Constant2 : Constant  Value=phirefVAS
  Demux : Demux  Outputs=2
  Gain1 : Gain  Gain=rVASmax
  Gain3 : Gain  Gain=phiScaleVAS
  Gain4 : Gain  Gain=rhoVAS/phiScaleVAS
  Gain5 : Gain  Gain=phiScaleVAS
  Mux : Mux  Inputs=2
  Sum1 : Sum  Inputs=-+
  Sum2 : Sum  Inputs=|+-
  Sum3 : Sum  Inputs=-+|
  Sum5 : Sum  Inputs=|+-
  length change term : Trigonometry
  offset correction term : Trigonometry
  variable lever term : Trigonometry  Operator=cos
  lmtu [m] : Outport
  lever [m] : Outport  Port=2
  wires:
  Constant/1 -> Sum5/1
  Sum5/1 -> lmtu [m]/1
  phi23 [rad]/1 -> Sum3/2
  Sum3/1 -> Gain3/1
  Constant1/1 -> Sum3/1, Sum2/2
  Sum2/1 -> Gain5/1
  Constant2/1 -> Sum2/1
  length change term/1 -> Sum1/2
  offset correction term/1 -> Sum1/1
  Sum1/1 -> Mux/1
  variable lever term/1 -> Mux/2
  Mux/1 -> Gain1/1
  Gain1/1 -> Demux/1
  Demux/2 -> lever [m]/1
  Demux/1 -> Gain4/1
  Gain3/1 -> variable lever term/1, length change term/1
  Gain5/1 -> offset correction term/1
  Gain4/1 -> Sum5/2

== system atrias_HW_boom_nmSt_kinSw_v2/Control/Behavior Control/Virtual Neuromuscular Control/Muscle Layer/VAS Link1 ==
  note: Muscle Length and Moment Arm
  phi23 [rad] : Inport
  Constant : Constant  Value=lslackVAS+loptVAS
  Constant1 : Constant  Value=phimaxVAS
  Constant2 : Constant  Value=phirefVAS
  Demux : Demux  Outputs=2
  Gain1 : Gain  Gain=rVASmax
  Gain3 : Gain  Gain=phiScaleVAS
  Gain4 : Gain  Gain=rhoVAS/phiScaleVAS
  Gain5 : Gain  Gain=phiScaleVAS
  Mux : Mux  Inputs=2
  Sum1 : Sum  Inputs=-+
  Sum2 : Sum  Inputs=|+-
  Sum3 : Sum  Inputs=-+|
  Sum5 : Sum  Inputs=|+-
  length change term : Trigonometry
  offset correction term : Trigonometry
  variable lever term : Trigonometry  Operator=cos
  lmtu [m] : Outport
  lever [m] : Outport  Port=2
  wires:
  Constant/1 -> Sum5/1
  Sum5/1 -> lmtu [m]/1
  phi23 [rad]/1 -> Sum3/2
  Sum3/1 -> Gain3/1
  Constant1/1 -> Sum3/1, Sum2/2
  Sum2/1 -> Gain5/1
  Constant2/1 -> Sum2/1
  length change term/1 -> Sum1/2
  offset correction term/1 -> Sum1/1
  Sum1/1 -> Mux/1
  variable lever term/1 -> Mux/2
  Mux/1 -> Gain1/1
  Gain1/1 -> Demux/1
  Demux/2 -> lever [m]/1
  Demux/1 -> Gain4/1
  Gain3/1 -> variable lever term/1, length change term/1
  Gain5/1 -> offset correction term/1
  Gain4/1 -> Sum5/2

== system atrias_HW_boom_nmSt_kinSw_v2/Control/Behavior Control/Virtual Neuromuscular Control/Muscle Layer/VAS1 ==
  note: SOLEUS Muscle-Tendon Dynamics
  note: Excitation Contraction Coupling
  STIM : Inport
  lmtc [m] : Inport  Port=2
  1 : Product  Inputs=**  SaturateOnIntegerOverflow=on  InputSameDT=on  OutDataTypeStr=Inherit: Same as first input
  1/lslack : Gain  Gain=1/lslackVAS  SaturateOnIntegerOverflow=on  OutDataTypeStr=Inherit: Same as input  ParamDataTypeStr=Inherit: Same as input
  BE force-length relation : Subsystem
  CE force-length relation : Subsystem
  CE inverse force-velocity relation : Subsystem
  Constant : Constant  Value=lslackVAS
  ECC TransferFcn : simulink_extras/Additional Linear/Transfer Fcn (with initial outputs)  N=[1]  D="[mtu_tau  1]"  Y0=mtu_preA  U0=0
      settings: AttributesFormatString=pre-activation: %<Y0>
  Fmax : Gain  Gain=FmaxVAS  SaturateOnIntegerOverflow=on  OutDataTypeStr=Inherit: Same as input  ParamDataTypeStr=Inherit: Same as input
  Fv = Fse / (A*Fce) : Product  Inputs=*/  SaturateOnIntegerOverflow=on  InputSameDT=on  OutDataTypeStr=Inherit: Same as first input
  Integrator : Integrator  InitialConditionSource=external  LowerSaturationLimit=0.05
  PE force-length relation : Subsystem
  SE force-length relation : Subsystem
  Saturation : Saturate  UpperLimit=1  LowerLimit=0.01
  Sum : Sum  Inputs=|+-  SaturateOnIntegerOverflow=on  InputSameDT=on  OutDataTypeStr=Inherit: Same as first input
  Sum2 : Sum  Inputs=|-+  SaturateOnIntegerOverflow=on  InputSameDT=on  OutDataTypeStr=Inherit: Same as first input
  Sum3 : Sum  SaturateOnIntegerOverflow=on  InputSameDT=on  OutDataTypeStr=Inherit: Same as first input
  Sum4 : Sum  SaturateOnIntegerOverflow=on  InputSameDT=on  OutDataTypeStr=Inherit: Same as first input
  lce/lopt : Gain  Gain=1/loptVAS  SaturateOnIntegerOverflow=on  OutDataTypeStr=Inherit: Same as input  ParamDataTypeStr=Inherit: Same as input
  vmax*lopt : Gain  Gain=vmaxVAS*loptVAS  SaturateOnIntegerOverflow=on  OutDataTypeStr=Inherit: Same as input  ParamDataTypeStr=Inherit: Same as input
  Fmtc : Outport  InitialOutput=0
  Lce : Outport  Port=2  InitialOutput=0
  Vce : Outport  Port=3  InitialOutput=0
  A : Outport  Port=4  InitialOutput=0
  wires:
  Integrator/1 -> Sum/2, lce/lopt/1, Lce/1  "lce"
  Sum/1 -> 1/lslack/1  "lse"
  lce/lopt/1 -> CE force-length relation/1(lce [lopt]), BE force-length relation/1(lce [lopt]), PE force-length relation/1(lce [lopt])
  Fv = Fse / (A*Fce)/1 -> CE inverse force-velocity relation/1(Fv[Fmax])  "fv"
  vmax*lopt/1 -> Integrator/1, Vce/1  "vce"
  lmtc [m]/1 -> Sum2/2, Sum/1  "lmtc"
  Fmax/1 -> Fmtc/1  "Fmtc"
  1/lslack/1 -> SE force-length relation/1(lse [lslack])
  SE force-length relation/1(fse [Fmax]) -> Fmax/1, Sum4/1
  Sum2/1 -> Integrator/2
  Constant/1 -> Sum2/1
  CE force-length relation/1(fce [Fmax]) -> 1/1
  Sum4/1 -> Fv = Fse / (A*Fce)/1
  PE force-length relation/1(fpe [Fmax]) -> Sum3/1
  1/1 -> Sum3/2
  BE force-length relation/1(fbe [Fmax]) -> Sum4/2
  Sum3/1 -> Fv = Fse / (A*Fce)/2
  CE inverse force-velocity relation/1(v[vmax]) -> vmax*lopt/1
  STIM/1 -> ECC TransferFcn/1
  ECC TransferFcn/1 -> Saturation/1
  Saturation/1 -> A/1, 1/2
